simulink model "mpc_pendcartImplicitMPC"  (R2019a)
settings: Solver=VariableStepAuto  StartTime=0.0  StopTime=10.0  RelTol=1e-3
values from neighbouring files (symbols this model uses):
  A = [0,1 ... (first row only)    [ControlOfAnInvertedPendulumOnACartExample.m]
  B = [0; (L/J)]    [ControlOfAnInvertedPendulumOnACartExample.m]
  GoalPos = [pi;0]    [ControlOfAnInvertedPendulumOnACartExample.m]
  K = place(A,B,p)    [ControlOfAnInvertedPendulumOnACartExample.m]
settings Model: Creator=Lucifer  LastModifiedBy=Lucifer

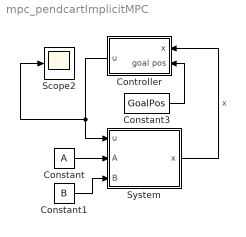
== system mpc_pendcartImplicitMPC ==
  "\tSystem" : Subsystem  AncestorBlock=cstblocks/Linear Parameter Varying/Varying State Space  mask(Varying State Space){x0=0, xNames='', OutputX=on, OutputDX=on}
      mask prompts: x0 "Control:simulink:VaryingSSLabel1"; xNames "Control:simulink:VaryingSSLabel2"; OutputX "Control:simulink:VaryingSSLabel3"; OutputDX "Control:simulink:VaryingSSLabel4"
      mask help: Control:simulink:VaryingSS1
      mask init:
      | % Use exact linearization of product block
      | % pblks = find_system(gcb,'FollowLinks','on',...
      | %    'LookUnderMasks','all','SearchDepth',1,'BlockType','Product');
      | % rep = struct(...
      | %    'Specification','controllib.internal.blocks.matrixProductJacobian',...
      | %    'Type','Function',...
      | %    'ParameterNames','',...
      | %    'ParameterValues','');
      | % for i=1:numel(pblks)
      | %    set_param(pblks{i},...
      | %       'SCDEnableBlockLinearizationSpecification','on',...
      | %       'SCDBlockLinearizationSpecification',rep)
      | % end
      | SimStatus = get_param(bdroot,'SimulationStatus');
      | if any(strcmp(SimStatus,{'initializing','updating','stopped'}))
      |    varyingBlockMask('ss',gcb,OutputX,OutputDX)
      | end
      mask Help: eval('ctrlguihelp(''VaryingSSCT'');')
      mask DialogControl x0 Prompt: Initial conditions:
      mask DialogControl xNames Prompt: State names (e.g., 'position'):
      mask DialogControl OutputX Prompt: Output states
      mask DialogControl OutputDX Prompt: Output state derivatives
      mask Display:
      | port_label('input', 1, 'u')
      | port_label('input', 2, 'A')
      | port_label('input', 3, 'B')
      | port_label('input', 4, 'C')
      | port_label('input', 5, 'D')
      | port_label('output', 1, 'y')
      | next_ = 2;
      | if OutputX
      |    port_label('output', next_, 'x')
      |    next_ = next_+1;
      | end
      | if OutputDX
      |    port_label('output', next_, 'dx')
      |    next_ = next_+1;
      | end
      | text(0.5,0.65,'dx = A x + B u',...
      |    'horizontalAlignment', 'center','texmode','on')
      | text(0.5,0.35,'y = C x + D u',...
      |    'horizontalAlignment', 'center','texmode','on')
  Constant : Constant  Value=A
  Constant1 : Constant  Value=B
  Constant3 : Constant  Value=GoalPos
  Controller : Subsystem
  Scope2 : Scope
  wires:
  Constant/1 -> "\tSystem"/2(A)
  Constant1/1 -> "\tSystem"/3(B)
  "\tSystem"/1(x) -> Controller/1(x)  "x"
  Controller/1(u) -> Scope2/1, "\tSystem"/1(u)
  Constant3/1 -> Controller/2(goal pos)

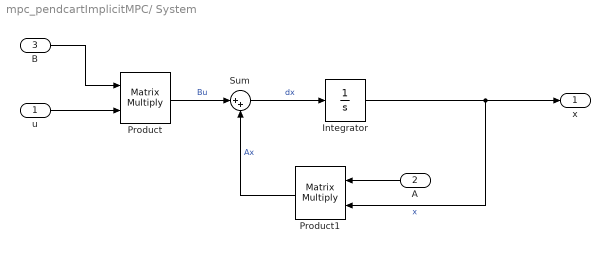
== system mpc_pendcartImplicitMPC/	System ==
  u : Inport  Unit=N
  A : Inport  Port=2
  B : Inport  Port=3
  Integrator : Integrator  InitialCondition=x0  ContinuousStateAttributes=xNames
  Product : Product  SCDEnableBlockLinearizationSpecification=on  Multiplication=Matrix(*)
  Product1 : Product  SCDEnableBlockLinearizationSpecification=on  Multiplication=Matrix(*)
  Sum : Sum  Inputs=|++
  x : Outport
  wires:
  u/1 -> Product/2
  A/1 -> Product1/1
  Product1/1 -> Sum/2  "Ax"
  B/1 -> Product/1
  Integrator/1 -> x/1, Product1/2  "x"
  Sum/1 -> Integrator/1  "dx"
  Product/1 -> Sum/1  "Bu"

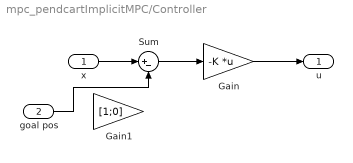
== system mpc_pendcartImplicitMPC/Controller ==
  x : Inport
  goal pos : Inport  Port=2
  Gain : Gain  Gain=-K  Multiplication=Matrix(K*u)
  Gain1 : Gain  Gain=[1;0]
  Sum : Sum  Inputs=|+-
  u : Outport
  wires:
  x/1 -> Sum/1
  Gain/1 -> u/1
  Sum/1 -> Gain/1
  goal pos/1 -> Sum/2
